simulink model "ES101A_DiagcMgrProxyX"  (R2013b)
settings: Solver=ode45  StartTime=0.0  StopTime=10.0  RelTol=1e-3
values from neighbouring files (symbols this model uses):
  DFTAGICNTR_CNT_U08 = DataDict.Constant    [ES101A_DiagcMgr_DataDict.m]
  DIAGCMGR_NTCINFOSTSTESTFAILD_CNT_U08 = DataDict.Constant    [ES101A_DiagcMgrProxyX_DataDict.m]    (also in ES101A_DiagcMgr_DataDict.m)
  DIAGCMGR_NTCINFOSTSTESTFAILDTHISIGNCYC_CNT_U08 = DataDict.Constant    [ES101A_DiagcMgr_DataDict.m]
  DIAGCMGR_NTCINFOSTSTESTNOTCMPLTHISIGNCYC_CNT_U08 = DataDict.Constant    [ES101A_DiagcMgrProxyX_DataDict.m]    (also in ES101A_DiagcMgr_DataDict.m)
  DiagcMgrFltResp = DataDict.Calibration    [ES101A_DiagcMgrProxyX_DataDict.m]    (also in ES101A_DiagcMgr_DataDict.m)
  DIAGCSTSDFTHWAG_CNT_U16 = DataDict.Constant    [ES101A_DiagcMgr_DataDict.m]
  DIAGCSTSDFTHWAGSERLCOMEXPRTVAL_CNT_U16 = DataDict.Constant    [ES101A_DiagcMgr_DataDict.m]
  DIAGCSTSDFTVEHSPD_CNT_U16 = DataDict.Constant    [ES101A_DiagcMgr_DataDict.m]
  DIAGCSTSININVAL_CNT_U16 = DataDict.Constant    [ES101A_DiagcMgrProxyX_DataDict.m]    (also in ES101A_DiagcMgr_DataDict.m)
  DIAGCSTSIVTR1INACTV_CNT_U16 = DataDict.Constant    [ES101A_DiagcMgr_DataDict.m]
  DIAGCSTSIVTR2INACTV_CNT_U16 = DataDict.Constant    [ES101A_DiagcMgr_DataDict.m]
  DIAGCSTSLIMDTPRFMNC_CNT_U16 = DataDict.Constant    [ES101A_DiagcMgr_DataDict.m]
  DIAGCSTSWHLIMBREJCTNDI_CNT_U16 = DataDict.Constant    [ES101A_DiagcMgr_DataDict.m]
  ELECGLBPRM_IVTRCNT_CNT_U08 = DataDict.ConfigParam    [ES101A_DiagcMgrProxyX_DataDict.m]    (also in ES101A_DiagcMgr_DataDict.m)
  MAXRAMPRATE_ULSPERSEC_F32 = DataDict.Constant    [ES101A_DiagcMgrProxyX_DataDict.m]    (also in ES101A_DiagcMgr_DataDict.m)
  MINRAMPRATE_ULSPERSEC_F32 = DataDict.Constant    [ES101A_DiagcMgrProxyX_DataDict.m]    (also in ES101A_DiagcMgr_DataDict.m)
  SCAMOTTQCMDTOONE_ULS_F32 = DataDict.Constant    [ES101A_DiagcMgrProxyX_DataDict.m]    (also in ES101A_DiagcMgr_DataDict.m)
  SCAMOTTQCMDTOZERO_ULS_F32 = DataDict.Constant    [ES101A_DiagcMgrProxyX_DataDict.m]    (also in ES101A_DiagcMgr_DataDict.m)
undefined symbols (not defined in the file or in its folder): ActvMotTqCmdSca, ActvRampRate, AgiCntr, DIAGCMGR_APPLIDXX_CNT_U08, DiagcMgrNtcMap, DiagcSts, NtcStInfo, Sts
libraries: simulink x21
(part 2 of 3)

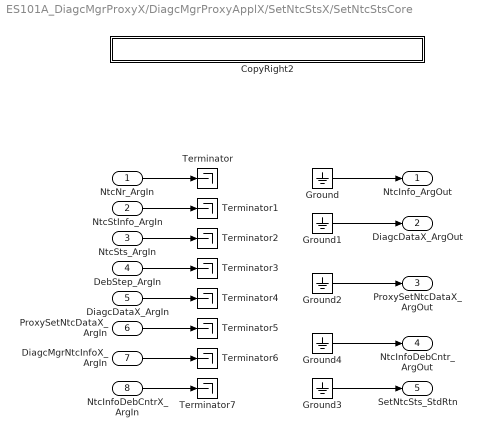
== system ES101A_DiagcMgrProxyX/DiagcMgrProxyApplX/SetNtcStsX/SetNtcStsCore ==
  NtcNr_ArgIn : Inport  OutDataTypeStr=Enum: NtcNr1
  NtcStInfo_ArgIn : Inport  Port=2
  NtcSts_ArgIn : Inport  Port=3
  DebStep_ArgIn : Inport  Port=4
  DiagcDataX_ArgIn : Inport  Port=5
  ProxySetNtcDataX_ArgIn : Inport  Port=6
  DiagcMgrNtcInfoX_ArgIn : Inport  Port=7
  NtcInfoDebCntrX_ArgIn : Inport  Port=8
  CopyRight2 : Subsystem  Description=|  mask(Copyright Information){none=on}
      | Copyright info block.                                               
      |                                                                     
      | Place copyright information at the top of every subsystem in design.
      mask prompts: none "No parameters"
      mask help: Place copyright information at the top of every subsystem in design.
      mask Display:
      | NxtrConf = 'Nexteer Confidential';
      | 
      | sys = bdroot; %handle for the current model ("system")
      | first = get_param(sys,'Created');
      | first = first(end-3:end);  %year is last four digits
      | 
      | last = get_param(sys,'LastModifiedDate');
      | if isempty(last)
      |     last = datestr(now,'yyyy');
      | else
      |     last = last(end-3:end);
      | end
      | 
      | if strcmp(first,last)
      |     fprintf('%s -- Copyright %s Nexteer',NxtrConf,first)
      | else
      |     fprintf('%s -- %s%s- %s Nexteer',NxtrConf,char(169),first,last)
      | end
  Ground{,1..4} (5 alike) : Ground
  Terminator{,1..7} (8 alike) : Terminator
  "NtcInfo_ArgOut " : Outport
  "DiagcDataX_ArgOut " : Outport  Port=2
  "ProxySetNtcDataX_ArgOut " : Outport  Port=3
  "NtcInfoDebCntr_ArgOut " : Outport  Port=4
  SetNtcSts_StdRtn : Outport  Port=5
  wires:
  NtcNr_ArgIn/1 -> Terminator/1
  NtcStInfo_ArgIn/1 -> Terminator1/1
  NtcSts_ArgIn/1 -> Terminator2/1
  DebStep_ArgIn/1 -> Terminator3/1
  DiagcDataX_ArgIn/1 -> Terminator4/1
  ProxySetNtcDataX_ArgIn/1 -> Terminator5/1
  DiagcMgrNtcInfoX_ArgIn/1 -> Terminator6/1
  NtcInfoDebCntrX_ArgIn/1 -> Terminator7/1
  Ground/1 -> "NtcInfo_ArgOut "/1
  Ground1/1 -> "DiagcDataX_ArgOut "/1
  Ground2/1 -> "ProxySetNtcDataX_ArgOut "/1
  Ground3/1 -> SetNtcSts_StdRtn/1
  Ground4/1 -> "NtcInfoDebCntr_ArgOut "/1

== system ES101A_DiagcMgrProxyX/DiagcMgrProxyApplX/DiagcMgrProxyApplXInit1/DiagcMgrIninCore/CopyRight2 ==

== system ES101A_DiagcMgrProxyX/DiagcMgrProxyApplX/DiagcMgrProxyApplXPer1/Clear All NTCs/CopyRight2 ==

== system ES101A_DiagcMgrProxyX/DiagcMgrProxyApplX/DiagcMgrProxyApplXPer1/Clear All NTCs/For Number of NTCs in NtcInfoAryX ==
  Number of Iterations : Inport
  Clear the NTCs that are active : Subsystem  RequirementInfo="{'linktype_rmi_doors' '0000c474 (/ESG Group/FDD Module Requirements/EA4 Specific/ES101A_DiagcMgr)' '#ES101A_298' 'true' 'REQ:  ES101A_298' '' ; 'linktype_rmi_doors' '0000c474 (/ESG Group/FDD Module Requirements/EA4 Specific/ES101A_DiagcMgr)' '#ES101A_185' 'true' 'REQ:  ES101A_185' '' ; 'linktype_rmi_doors' '0000c474 (/ESG Group/FDD Module Requirements/EA4 Specific/ES101A_DiagcMgr)' '#ES101A_256' 'true' 'REQ:  ES101A_256' '' ; 'linktype_rmi_doors' '0000c474 (/ESG Group/FDD Module Requirements/EA4 Specific/ES101A_DiagcMgr)' '#ES101A_255' 'true' 'REQ:  ES101A_255' '' ; 'linktype_rmi_doors' '0000c474 (/ESG Group/FDD Module Requirements/EA4 Specific/ES101A_DiagcMgr)' '#ES101A_254' 'true' 'REQ:  ES101A_254' '' ; 'linktype_rmi_doors' '0000c474 (/ESG Group/FDD Module Requirements/EA4 Specific/ES101A_DiagcMgr)' '#ES101A_297' 'true' 'REQ:  ES101A_297' '' ; 'linktype_rmi_doors' '0000c474 (/ESG Group/FDD Module Requirements/EA4 Specific/ES101A_DiagcMgr)' '#ES101A_305' 'true' 'REQ:  ES101A_305' '' } %GIDa_e344900f_fb8d_4798_8862_4b0202a8bbef"
  CopyRight2 : Subsystem  Description=|  mask(Copyright Information){none=on}
      | Copyright info block.                                               
      |                                                                     
      | Place copyright information at the top of every subsystem in design.
      mask prompts: none "No parameters"
      mask help: Place copyright information at the top of every subsystem in design.
      mask Display:
      | NxtrConf = 'Nexteer Confidential';
      | 
      | sys = bdroot; %handle for the current model ("system")
      | first = get_param(sys,'Created');
      | first = first(end-3:end);  %year is last four digits
      | 
      | last = get_param(sys,'LastModifiedDate');
      | if isempty(last)
      |     last = datestr(now,'yyyy');
      | else
      |     last = last(end-3:end);
      | end
      | 
      | if strcmp(first,last)
      |     fprintf('%s -- Copyright %s Nexteer',NxtrConf,first)
      | else
      |     fprintf('%s -- %s%s- %s Nexteer',NxtrConf,char(169),first,last)
      | end
  For Iterator : ForIterator  IterationSource=external  IterationLimit=255  IndexMode=Zero-based  IterationVariableDataType=int8
  wires:
  For Iterator/1 -> Clear the NTCs that are active/1(NtcInfoIdx)
  Number of Iterations/1 -> For Iterator/1

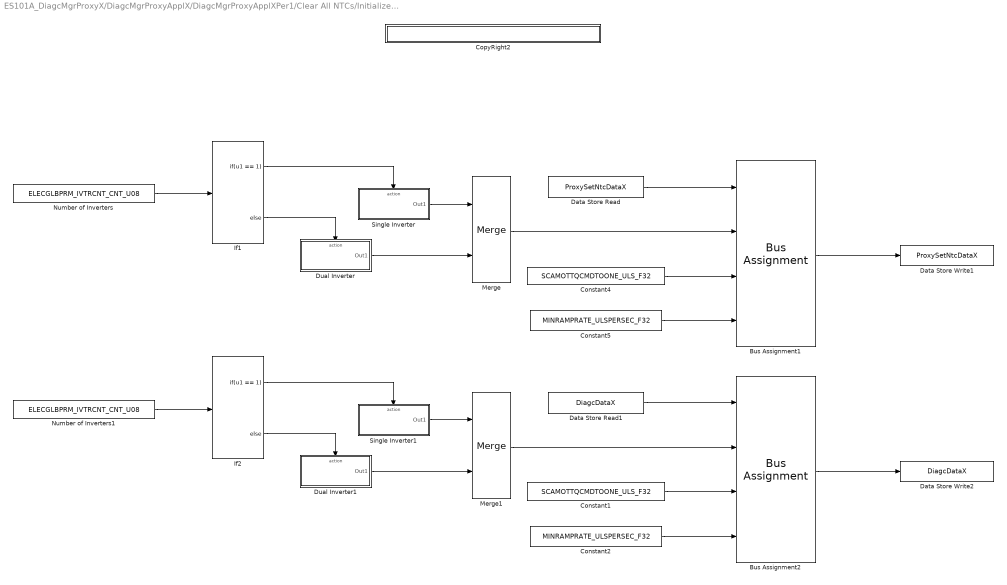
== system ES101A_DiagcMgrProxyX/DiagcMgrProxyApplX/DiagcMgrProxyApplXPer1/Clear All NTCs/Initialize Proxy SetNtc and DiagcData values ==
  Bus Assignment1 : BusAssignment  AssignedSignals=DiagcSts,ActvRampRate,ActvMotTqCmdSca
  Bus Assignment2 : BusAssignment  AssignedSignals=DiagcSts,ActvRampRate,ActvMotTqCmdSca
  Constant1 : Constant  Value=SCAMOTTQCMDTOONE_ULS_F32  OutDataTypeStr=single
  Constant2 : Constant  Value=MINRAMPRATE_ULSPERSEC_F32  OutDataTypeStr=single
  Constant4 : Constant  Value=SCAMOTTQCMDTOONE_ULS_F32  OutDataTypeStr=single
  Constant5 : Constant  Value=MINRAMPRATE_ULSPERSEC_F32  OutDataTypeStr=single
  CopyRight2 : Subsystem  Description=|  mask(Copyright Information){none=on}
      | Copyright info block.                                               
      |                                                                     
      | Place copyright information at the top of every subsystem in design.
      mask prompts: none "No parameters"
      mask help: Place copyright information at the top of every subsystem in design.
      mask Display:
      | NxtrConf = 'Nexteer Confidential';
      | 
      | sys = bdroot; %handle for the current model ("system")
      | first = get_param(sys,'Created');
      | first = first(end-3:end);  %year is last four digits
      | 
      | last = get_param(sys,'LastModifiedDate');
      | if isempty(last)
      |     last = datestr(now,'yyyy');
      | else
      |     last = last(end-3:end);
      | end
      | 
      | if strcmp(first,last)
      |     fprintf('%s -- Copyright %s Nexteer',NxtrConf,first)
      | else
      |     fprintf('%s -- %s%s- %s Nexteer',NxtrConf,char(169),first,last)
      | end
  Data Store Read : DataStoreRead  DataStoreName=ProxySetNtcDataX
  Data Store Read1 : DataStoreRead  DataStoreName=DiagcDataX
  Data Store Write1 : DataStoreWrite  DataStoreName=ProxySetNtcDataX
  Data Store Write2 : DataStoreWrite  DataStoreName=DiagcDataX
  Dual Inverter : Subsystem  TreatAsAtomicUnit=on
  Dual Inverter1 : Subsystem  TreatAsAtomicUnit=on
  If1 : If  IfExpression=u1 == 1
  If2 : If  IfExpression=u1 == 1
  Merge : Merge
  Merge1 : Merge
  Number of Inverters : Constant  Value=ELECGLBPRM_IVTRCNT_CNT_U08
  Number of Inverters1 : Constant  Value=ELECGLBPRM_IVTRCNT_CNT_U08
  Single Inverter : Subsystem  TreatAsAtomicUnit=on
  Single Inverter1 : Subsystem  TreatAsAtomicUnit=on
  wires:
  Data Store Read/1 -> Bus Assignment1/1
  Bus Assignment1/1 -> Data Store Write1/1
  Constant4/1 -> Bus Assignment1/3
  Constant5/1 -> Bus Assignment1/4
  Merge/1 -> Bus Assignment1/2
  If1/2 -> Dual Inverter/Action
  If1/1 -> Single Inverter/Action
  Number of Inverters/1 -> If1/1
  Dual Inverter/1(Out1) -> Merge/2
  Single Inverter/1(Out1) -> Merge/1
  Data Store Read1/1 -> Bus Assignment2/1
  Bus Assignment2/1 -> Data Store Write2/1
  Constant1/1 -> Bus Assignment2/3
  Constant2/1 -> Bus Assignment2/4
  Merge1/1 -> Bus Assignment2/2
  If2/2 -> Dual Inverter1/Action
  If2/1 -> Single Inverter1/Action
  Number of Inverters1/1 -> If2/1
  Dual Inverter1/1(Out1) -> Merge1/2
  Single Inverter1/1(Out1) -> Merge1/1

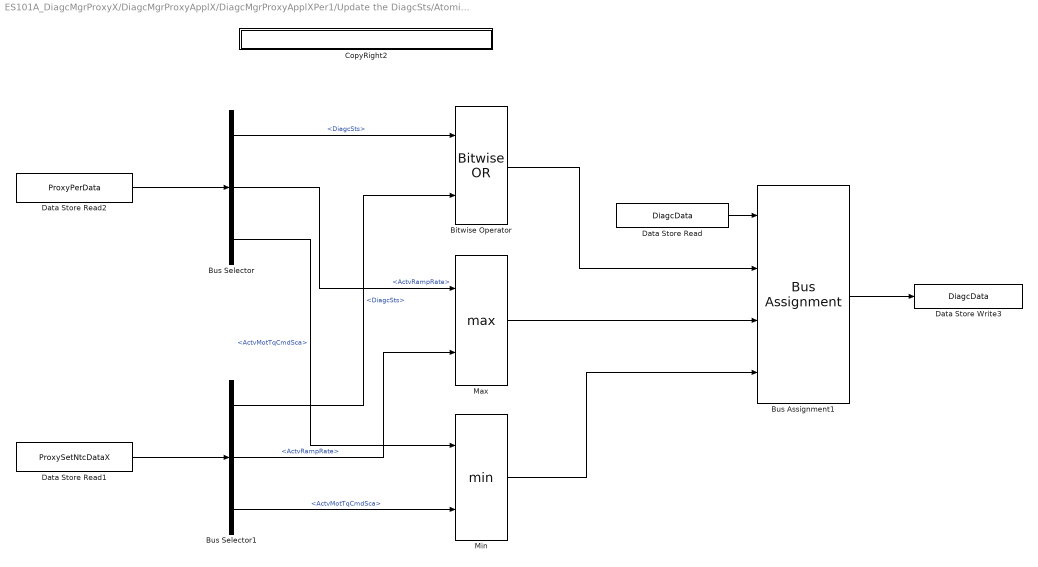
== system ES101A_DiagcMgrProxyX/DiagcMgrProxyApplX/DiagcMgrProxyApplXPer1/Update the DiagcSts/Atomic Section ==
  Bitwise Operator : simulink/Logic and Bit Operations/Bitwise Operator  logicop=OR  UseBitMask=off  NumInputPorts=2  BitMask=bin2dec('11011001')  BitMaskRealWorld=Stored Integer
  Bus Assignment1 : BusAssignment  AssignedSignals=DiagcSts,ActvRampRate,ActvMotTqCmdSca
  Bus Selector : BusSelector  OutputSignals=DiagcSts,ActvRampRate,ActvMotTqCmdSca
  Bus Selector1 : BusSelector  OutputSignals=DiagcSts,ActvRampRate,ActvMotTqCmdSca
  CopyRight2 : Subsystem  Description=|  mask(Copyright Information){none=on}
      | Copyright info block.                                               
      |                                                                     
      | Place copyright information at the top of every subsystem in design.
      mask prompts: none "No parameters"
      mask help: Place copyright information at the top of every subsystem in design.
      mask Display:
      | NxtrConf = 'Nexteer Confidential';
      | 
      | sys = bdroot; %handle for the current model ("system")
      | first = get_param(sys,'Created');
      | first = first(end-3:end);  %year is last four digits
      | 
      | last = get_param(sys,'LastModifiedDate');
      | if isempty(last)
      |     last = datestr(now,'yyyy');
      | else
      |     last = last(end-3:end);
      | end
      | 
      | if strcmp(first,last)
      |     fprintf('%s -- Copyright %s Nexteer',NxtrConf,first)
      | else
      |     fprintf('%s -- %s%s- %s Nexteer',NxtrConf,char(169),first,last)
      | end
  Data Store Read : DataStoreRead  DataStoreName=DiagcData  DataStoreElements=DiagcData
  Data Store Read1 : DataStoreRead  DataStoreName=ProxySetNtcDataX
  Data Store Read2 : DataStoreRead  DataStoreName=ProxyPerData
  Data Store Write3 : DataStoreWrite  DataStoreName=DiagcData  DataStoreElements=DiagcData
  Max : MinMax  Function=max  Inputs=2
  Min : MinMax  Inputs=2
  wires:
  Bus Selector/3 -> Min/1  "<ActvMotTqCmdSca>"
  Bus Selector1/3 -> Min/2  "<ActvMotTqCmdSca>"
  Bus Selector/2 -> Max/1  "<ActvRampRate>"
  Bus Selector1/2 -> Max/2  "<ActvRampRate>"
  Bus Selector/1 -> Bitwise Operator/1  "<DiagcSts>"
  Bus Selector1/1 -> Bitwise Operator/2  "<DiagcSts>"
  Data Store Read2/1 -> Bus Selector/1
  Data Store Read1/1 -> Bus Selector1/1
  Bus Assignment1/1 -> Data Store Write3/1
  Bitwise Operator/1 -> Bus Assignment1/2
  Max/1 -> Bus Assignment1/3
  Min/1 -> Bus Assignment1/4
  Data Store Read/1 -> Bus Assignment1/1

== system ES101A_DiagcMgrProxyX/DiagcMgrProxyApplX/DiagcMgrProxyApplXPer1/Update the DiagcSts/CopyRight2 ==

== system ES101A_DiagcMgrProxyX/DiagcMgrProxyApplX/DiagcMgrProxyApplXPer1/Update the DiagcSts/For Number of NTCs ==
  Number of Iterations : Inport
  Bus Selector2 : BusSelector  OutputSignals=Sts
  CopyRight2 : Subsystem  Description=|  mask(Copyright Information){none=on}
      | Copyright info block.                                               
      |                                                                     
      | Place copyright information at the top of every subsystem in design.
      mask prompts: none "No parameters"
      mask help: Place copyright information at the top of every subsystem in design.
      mask Display:
      | NxtrConf = 'Nexteer Confidential';
      | 
      | sys = bdroot; %handle for the current model ("system")
      | first = get_param(sys,'Created');
      | first = first(end-3:end);  %year is last four digits
      | 
      | last = get_param(sys,'LastModifiedDate');
      | if isempty(last)
      |     last = datestr(now,'yyyy');
      | else
      |     last = last(end-3:end);
      | end
      | 
      | if strcmp(first,last)
      |     fprintf('%s -- Copyright %s Nexteer',NxtrConf,first)
      | else
      |     fprintf('%s -- %s%s- %s Nexteer',NxtrConf,char(169),first,last)
      | end
  Data Store Read1 : DataStoreRead  DataStoreName=NtcNrAryApplX
  Data Store Read2 : DataStoreRead  DataStoreName=DiagcMgrNtcInfoXAry
  For Iterator : ForIterator  IterationSource=external  IndexMode=Zero-based
  Selector1 : Selector  IndexMode=Zero-based  InputPortWidth=1  IndexOptions=Index vector (port)  Indices=[1 3]  OutputSizes=1
  Selector2 : Selector  IndexMode=Zero-based  InputPortWidth=1  IndexOptions=Index vector (port)  Indices=[1 3]  OutputSizes=1
  Update DiagcSts and Ramp Response : Subsystem  TreatAsAtomicUnit=on
  wires:
  Number of Iterations/1 -> For Iterator/1
  For Iterator/1 -> Selector2/2, Selector1/2
  Selector1/1 -> Bus Selector2/1
  Data Store Read2/1 -> Selector1/1
  Bus Selector2/1 -> Update DiagcSts and Ramp Response/1(Sts)  "<Sts>"
  Data Store Read1/1 -> Selector2/1
  Selector2/1 -> Update DiagcSts and Ramp Response/2(NtcNr)

== system ES101A_DiagcMgrProxyX/DiagcMgrProxyApplX/DiagcMgrProxyApplXPer1/Update the DiagcSts/Initialize Proxy Per values ==
  Bus Assignment1 : BusAssignment  AssignedSignals=DiagcSts,ActvRampRate,ActvMotTqCmdSca
  Constant4 : Constant  Value=SCAMOTTQCMDTOONE_ULS_F32  OutDataTypeStr=single
  Constant5 : Constant  Value=MINRAMPRATE_ULSPERSEC_F32  OutDataTypeStr=single
  CopyRight2 : Subsystem  Description=|  mask(Copyright Information){none=on}
      | Copyright info block.                                               
      |                                                                     
      | Place copyright information at the top of every subsystem in design.
      mask prompts: none "No parameters"
      mask help: Place copyright information at the top of every subsystem in design.
      mask Display:
      | NxtrConf = 'Nexteer Confidential';
      | 
      | sys = bdroot; %handle for the current model ("system")
      | first = get_param(sys,'Created');
      | first = first(end-3:end);  %year is last four digits
      | 
      | last = get_param(sys,'LastModifiedDate');
      | if isempty(last)
      |     last = datestr(now,'yyyy');
      | else
      |     last = last(end-3:end);
      | end
      | 
      | if strcmp(first,last)
      |     fprintf('%s -- Copyright %s Nexteer',NxtrConf,first)
      | else
      |     fprintf('%s -- %s%s- %s Nexteer',NxtrConf,char(169),first,last)
      | end
  Data Store Read : DataStoreRead  DataStoreName=ProxyPerData
  Data Store Write1 : DataStoreWrite  DataStoreName=ProxyPerData
  Dual Inverter : Subsystem  TreatAsAtomicUnit=on
  If1 : If  IfExpression=u1 == 1
  Merge : Merge
  Number of Inverters : Constant  Value=ELECGLBPRM_IVTRCNT_CNT_U08
  Single Inverter : Subsystem  TreatAsAtomicUnit=on
  wires:
  Data Store Read/1 -> Bus Assignment1/1
  Bus Assignment1/1 -> Data Store Write1/1
  Constant4/1 -> Bus Assignment1/3
  Constant5/1 -> Bus Assignment1/4
  Merge/1 -> Bus Assignment1/2
  If1/2 -> Dual Inverter/Action
  If1/1 -> Single Inverter/Action
  Number of Inverters/1 -> If1/1
  Dual Inverter/1(Out1) -> Merge/2
  Single Inverter/1(Out1) -> Merge/1

== system ES101A_DiagcMgrProxyX/DiagcMgrProxyApplX/DiagcMgrProxyApplXPer1/Update the DiagcSts/Initialize Proxy SetNtc values ==
  Bus Assignment1 : BusAssignment  AssignedSignals=DiagcSts,ActvRampRate,ActvMotTqCmdSca
  Constant4 : Constant  Value=SCAMOTTQCMDTOONE_ULS_F32  OutDataTypeStr=single
  Constant5 : Constant  Value=MINRAMPRATE_ULSPERSEC_F32  OutDataTypeStr=single
  CopyRight2 : Subsystem  Description=|  mask(Copyright Information){none=on}
      | Copyright info block.                                               
      |                                                                     
      | Place copyright information at the top of every subsystem in design.
      mask prompts: none "No parameters"
      mask help: Place copyright information at the top of every subsystem in design.
      mask Display:
      | NxtrConf = 'Nexteer Confidential';
      | 
      | sys = bdroot; %handle for the current model ("system")
      | first = get_param(sys,'Created');
      | first = first(end-3:end);  %year is last four digits
      | 
      | last = get_param(sys,'LastModifiedDate');
      | if isempty(last)
      |     last = datestr(now,'yyyy');
      | else
      |     last = last(end-3:end);
      | end
      | 
      | if strcmp(first,last)
      |     fprintf('%s -- Copyright %s Nexteer',NxtrConf,first)
      | else
      |     fprintf('%s -- %s%s- %s Nexteer',NxtrConf,char(169),first,last)
      | end
  Data Store Read : DataStoreRead  DataStoreName=ProxySetNtcDataX
  Data Store Write1 : DataStoreWrite  DataStoreName=ProxySetNtcDataX
  Dual Inverter : Subsystem  TreatAsAtomicUnit=on
  If1 : If  IfExpression=u1 == 1
  Merge : Merge
  Number of Inverters : Constant  Value=ELECGLBPRM_IVTRCNT_CNT_U08
  Single Inverter : Subsystem  TreatAsAtomicUnit=on
  wires:
  Data Store Read/1 -> Bus Assignment1/1
  Bus Assignment1/1 -> Data Store Write1/1
  Constant4/1 -> Bus Assignment1/3
  Constant5/1 -> Bus Assignment1/4
  Merge/1 -> Bus Assignment1/2
  If1/2 -> Dual Inverter/Action
  If1/1 -> Single Inverter/Action
  Number of Inverters/1 -> If1/1
  Dual Inverter/1(Out1) -> Merge/2
  Single Inverter/1(Out1) -> Merge/1

== system ES101A_DiagcMgrProxyX/DiagcMgrProxyApplX/GetNtcActvX/GetNtcActvCore/CopyRight2 ==

== system ES101A_DiagcMgrProxyX/DiagcMgrProxyApplX/GetNtcQlfrStsX/GetNtcQlfrStsCore/CopyRight2 ==

== system ES101A_DiagcMgrProxyX/DiagcMgrProxyApplX/GetNtcStsX/GetNtcStsCore/CopyRight2 ==

== system ES101A_DiagcMgrProxyX/DiagcMgrProxyApplX/SetNtcStsX/SetNtcStsCore/CopyRight2 ==

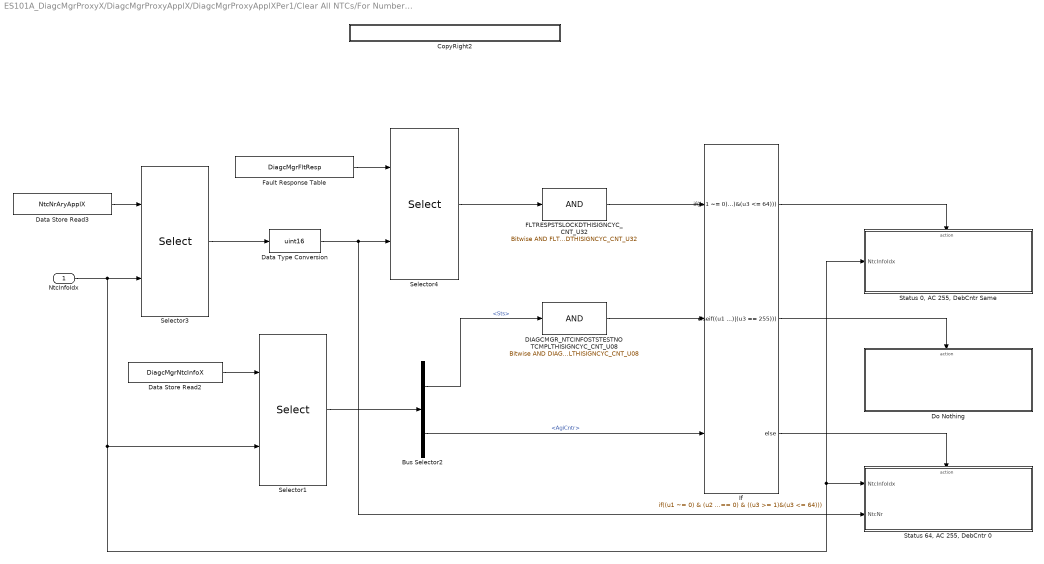
== system ES101A_DiagcMgrProxyX/DiagcMgrProxyApplX/DiagcMgrProxyApplXPer1/Clear All NTCs/For Number of NTCs in NtcInfoAryX/Clear the NTCs that are active ==
  NtcInfoIdx : Inport
  Bus Selector2 : BusSelector  OutputSignals=Sts,AgiCntr
  CopyRight2 : Subsystem  Description=|  mask(Copyright Information){none=on}
      | Copyright info block.                                               
      |                                                                     
      | Place copyright information at the top of every subsystem in design.
      mask prompts: none "No parameters"
      mask help: Place copyright information at the top of every subsystem in design.
      mask Display:
      | NxtrConf = 'Nexteer Confidential';
      | 
      | sys = bdroot; %handle for the current model ("system")
      | first = get_param(sys,'Created');
      | first = first(end-3:end);  %year is last four digits
      | 
      | last = get_param(sys,'LastModifiedDate');
      | if isempty(last)
      |     last = datestr(now,'yyyy');
      | else
      |     last = last(end-3:end);
      | end
      | 
      | if strcmp(first,last)
      |     fprintf('%s -- Copyright %s Nexteer',NxtrConf,first)
      | else
      |     fprintf('%s -- %s%s- %s Nexteer',NxtrConf,char(169),first,last)
      | end
  DIAGCMGR_NTCINFOSTSTESTNOTCMPLTHISIGNCYC_CNT_U08 : simulink/Logic and Bit Operations/Bitwise Operator  logicop=AND  UseBitMask=on  BitMask=DIAGCMGR_NTCINFOSTSTESTNOTCMPLTHISIGNCYC_CNT_U08  BitMaskRealWorld=Stored Integer
  Data Store Read2 : DataStoreRead  DataStoreName=DiagcMgrNtcInfoX
  Data Store Read3 : DataStoreRead  DataStoreName=NtcNrAryApplX
  Data Type Conversion : DataTypeConversion  OutDataTypeStr=uint16
  Do Nothing : Subsystem  TreatAsAtomicUnit=on
  FLTRESPSTSLOCKDTHISIGNCYC_CNT_U32 : simulink/Logic and Bit Operations/Bitwise Operator  RequirementInfo={} %GIDa_3c8fd334_aaa1_4aae_92b3_7b41709ff7dc  logicop=AND  UseBitMask=on  BitMask=FLTRESPSTSLOCKDTHISIGNCYC_CNT_U32  BitMaskRealWorld=Stored Integer
  Fault Response Table : Constant  Value=DiagcMgrFltResp
  If : If  NumInputs=3  IfExpression=(u1 ~= 0) & (u2 == 0) & ((u3 >= 1)&(u3 <= 64))  ElseIfExpressions=(u1 ~= 0) & (u2 == 0) & ((u3 == 0)|(u3 == 255))
  Selector1 : Selector  IndexMode=Zero-based  InputPortWidth=512  IndexOptions=Index vector (port)  Indices=[1 3]  OutputSizes=1
  Selector3 : Selector  IndexMode=Zero-based  InputPortWidth=22  IndexOptions=Index vector (port)  Indices=[1 3]  OutputSizes=1
  Selector4 : Selector  IndexMode=Zero-based  InputPortWidth=512  IndexOptions=Index vector (port)  Indices=[1 3]  OutputSizes=1
  "Status 0, AC 255, DebCntr Same" : Subsystem  TreatAsAtomicUnit=on
  "Status 64, AC 255, DebCntr 0" : Subsystem
  wires:
  Data Store Read3/1 -> Selector3/1
  Selector3/1 -> Data Type Conversion/1
  Fault Response Table/1 -> Selector4/1
  Selector4/1 -> FLTRESPSTSLOCKDTHISIGNCYC_CNT_U32/1
  FLTRESPSTSLOCKDTHISIGNCYC_CNT_U32/1 -> If/1
  Selector1/1 -> Bus Selector2/1
  Data Store Read2/1 -> Selector1/1
  Bus Selector2/1 -> DIAGCMGR_NTCINFOSTSTESTNOTCMPLTHISIGNCYC_CNT_U08/1  "<Sts>"
  Bus Selector2/2 -> If/3  "<AgiCntr>"
  DIAGCMGR_NTCINFOSTSTESTNOTCMPLTHISIGNCYC_CNT_U08/1 -> If/2
  Data Type Conversion/1 -> "Status 64, AC 255, DebCntr 0"/2(NtcNr), Selector4/2
  NtcInfoIdx/1 -> Selector3/2, "Status 0, AC 255, DebCntr Same"/1(NtcInfoIdx), "Status 64, AC 255, DebCntr 0"/1(NtcInfoIdx), Selector1/2
  If/3 -> "Status 64, AC 255, DebCntr 0"/Action
  If/2 -> Do Nothing/Action
  If/1 -> "Status 0, AC 255, DebCntr Same"/Action

== system ES101A_DiagcMgrProxyX/DiagcMgrProxyApplX/DiagcMgrProxyApplXPer1/Clear All NTCs/For Number of NTCs in NtcInfoAryX/CopyRight2 ==

== system ES101A_DiagcMgrProxyX/DiagcMgrProxyApplX/DiagcMgrProxyApplXPer1/Clear All NTCs/Initialize Proxy SetNtc and DiagcData values/CopyRight2 ==

== system ES101A_DiagcMgrProxyX/DiagcMgrProxyApplX/DiagcMgrProxyApplXPer1/Clear All NTCs/Initialize Proxy SetNtc and DiagcData values/Dual Inverter ==
  Action Port : ActionPort
  CopyRight2 : Subsystem  Description=|  mask(Copyright Information){none=on}
      | Copyright info block.                                               
      |                                                                     
      | Place copyright information at the top of every subsystem in design.
      mask prompts: none "No parameters"
      mask help: Place copyright information at the top of every subsystem in design.
      mask Display:
      | NxtrConf = 'Nexteer Confidential';
      | 
      | sys = bdroot; %handle for the current model ("system")
      | first = get_param(sys,'Created');
      | first = first(end-3:end);  %year is last four digits
      | 
      | last = get_param(sys,'LastModifiedDate');
      | if isempty(last)
      |     last = datestr(now,'yyyy');
      | else
      |     last = last(end-3:end);
      | end
      | 
      | if strcmp(first,last)
      |     fprintf('%s -- Copyright %s Nexteer',NxtrConf,first)
      | else
      |     fprintf('%s -- %s%s- %s Nexteer',NxtrConf,char(169),first,last)
      | end
  Inverter 2 Inactive : Constant  Value=0  OutDataTypeStr=uint16
  Out1 : Outport
  wires:
  Inverter 2 Inactive/1 -> Out1/1

== system ES101A_DiagcMgrProxyX/DiagcMgrProxyApplX/DiagcMgrProxyApplXPer1/Clear All NTCs/Initialize Proxy SetNtc and DiagcData values/Dual Inverter1 ==
  Action Port : ActionPort
  CopyRight2 : Subsystem  Description=|  mask(Copyright Information){none=on}
      | Copyright info block.                                               
      |                                                                     
      | Place copyright information at the top of every subsystem in design.
      mask prompts: none "No parameters"
      mask help: Place copyright information at the top of every subsystem in design.
      mask Display:
      | NxtrConf = 'Nexteer Confidential';
      | 
      | sys = bdroot; %handle for the current model ("system")
      | first = get_param(sys,'Created');
      | first = first(end-3:end);  %year is last four digits
      | 
      | last = get_param(sys,'LastModifiedDate');
      | if isempty(last)
      |     last = datestr(now,'yyyy');
      | else
      |     last = last(end-3:end);
      | end
      | 
      | if strcmp(first,last)
      |     fprintf('%s -- Copyright %s Nexteer',NxtrConf,first)
      | else
      |     fprintf('%s -- %s%s- %s Nexteer',NxtrConf,char(169),first,last)
      | end
  Inverter 2 Inactive : Constant  Value=0  OutDataTypeStr=uint16
  Out1 : Outport
  wires:
  Inverter 2 Inactive/1 -> Out1/1

== system ES101A_DiagcMgrProxyX/DiagcMgrProxyApplX/DiagcMgrProxyApplXPer1/Clear All NTCs/Initialize Proxy SetNtc and DiagcData values/Single Inverter ==
  Action Port : ActionPort
  CopyRight2 : Subsystem  Description=|  mask(Copyright Information){none=on}
      | Copyright info block.                                               
      |                                                                     
      | Place copyright information at the top of every subsystem in design.
      mask prompts: none "No parameters"
      mask help: Place copyright information at the top of every subsystem in design.
      mask Display:
      | NxtrConf = 'Nexteer Confidential';
      | 
      | sys = bdroot; %handle for the current model ("system")
      | first = get_param(sys,'Created');
      | first = first(end-3:end);  %year is last four digits
      | 
      | last = get_param(sys,'LastModifiedDate');
      | if isempty(last)
      |     last = datestr(now,'yyyy');
      | else
      |     last = last(end-3:end);
      | end
      | 
      | if strcmp(first,last)
      |     fprintf('%s -- Copyright %s Nexteer',NxtrConf,first)
      | else
      |     fprintf('%s -- %s%s- %s Nexteer',NxtrConf,char(169),first,last)
      | end
  Inverter 2 Inactive : Constant  Value=DIAGCSTSIVTR2INACTV_CNT_U16  OutDataTypeStr=uint16
  Out1 : Outport
  wires:
  Inverter 2 Inactive/1 -> Out1/1

== system ES101A_DiagcMgrProxyX/DiagcMgrProxyApplX/DiagcMgrProxyApplXPer1/Clear All NTCs/Initialize Proxy SetNtc and DiagcData values/Single Inverter1 ==
  Action Port : ActionPort
  CopyRight2 : Subsystem  Description=|  mask(Copyright Information){none=on}
      | Copyright info block.                                               
      |                                                                     
      | Place copyright information at the top of every subsystem in design.
      mask prompts: none "No parameters"
      mask help: Place copyright information at the top of every subsystem in design.
      mask Display:
      | NxtrConf = 'Nexteer Confidential';
      | 
      | sys = bdroot; %handle for the current model ("system")
      | first = get_param(sys,'Created');
      | first = first(end-3:end);  %year is last four digits
      | 
      | last = get_param(sys,'LastModifiedDate');
      | if isempty(last)
      |     last = datestr(now,'yyyy');
      | else
      |     last = last(end-3:end);
      | end
      | 
      | if strcmp(first,last)
      |     fprintf('%s -- Copyright %s Nexteer',NxtrConf,first)
      | else
      |     fprintf('%s -- %s%s- %s Nexteer',NxtrConf,char(169),first,last)
      | end
  Inverter 2 Inactive : Constant  Value=DIAGCSTSIVTR2INACTV_CNT_U16  OutDataTypeStr=uint16
  Out1 : Outport
  wires:
  Inverter 2 Inactive/1 -> Out1/1

== system ES101A_DiagcMgrProxyX/DiagcMgrProxyApplX/DiagcMgrProxyApplXPer1/Update the DiagcSts/Atomic Section/CopyRight2 ==

== system ES101A_DiagcMgrProxyX/DiagcMgrProxyApplX/DiagcMgrProxyApplXPer1/Update the DiagcSts/For Number of NTCs/CopyRight2 ==

== system ES101A_DiagcMgrProxyX/DiagcMgrProxyApplX/DiagcMgrProxyApplXPer1/Update the DiagcSts/For Number of NTCs/Update DiagcSts and Ramp Response ==
  Sts : Inport
  NtcNr : Inport  Port=2
  Bitwise Operator : simulink/Logic and Bit Operations/Bitwise Operator  logicop=AND  UseBitMask=off  NumInputPorts=2  BitMask=bin2dec('11011001')  BitMaskRealWorld=Stored Integer
  Bitwise Operator1 : simulink/Logic and Bit Operations/Bitwise Operator  logicop=AND  UseBitMask=off  NumInputPorts=2  BitMask=bin2dec('11011001')  BitMaskRealWorld=Stored Integer
  CopyRight2 : Subsystem  Description=|  mask(Copyright Information){none=on}
      | Copyright info block.                                               
      |                                                                     
      | Place copyright information at the top of every subsystem in design.
      mask prompts: none "No parameters"
      mask help: Place copyright information at the top of every subsystem in design.
      mask Display:
      | NxtrConf = 'Nexteer Confidential';
      | 
      | sys = bdroot; %handle for the current model ("system")
      | first = get_param(sys,'Created');
      | first = first(end-3:end);  %year is last four digits
      | 
      | last = get_param(sys,'LastModifiedDate');
      | if isempty(last)
      |     last = datestr(now,'yyyy');
      | else
      |     last = last(end-3:end);
      | end
      | 
      | if strcmp(first,last)
      |     fprintf('%s -- Copyright %s Nexteer',NxtrConf,first)
      | else
      |     fprintf('%s -- %s%s- %s Nexteer',NxtrConf,char(169),first,last)
      | end
  Do Nothing : Subsystem  TreatAsAtomicUnit=on
  If : If  IfExpression=u1 == 1
  Logical Operator : Logic  AllPortsSameDT=off  OutDataTypeStr=boolean
  NTC Test Failed Bit : Constant  Value=DIAGCMGR_NTCINFOSTSTESTFAILD_CNT_U08
  NTC Test Failed This Ignition Cycle Bit : Constant  Value=DIAGCMGR_NTCINFOSTSTESTFAILDTHISIGNCYC_CNT_U08
  Update Latest Values : Subsystem  TreatAsAtomicUnit=on
  wires:
  NtcNr/1 -> Update Latest Values/1(NtcNr)
  NTC Test Failed Bit/1 -> Bitwise Operator/1
  If/2 -> Do Nothing/Action
  If/1 -> Update Latest Values/Action
  NTC Test Failed This Ignition Cycle Bit/1 -> Bitwise Operator1/1
  Sts/1 -> Bitwise Operator/2, Bitwise Operator1/2
  Logical Operator/1 -> If/1
  Bitwise Operator1/1 -> Logical Operator/1
  Bitwise Operator/1 -> Logical Operator/2

== system ES101A_DiagcMgrProxyX/DiagcMgrProxyApplX/DiagcMgrProxyApplXPer1/Update the DiagcSts/Initialize Proxy Per values/CopyRight2 ==

== system ES101A_DiagcMgrProxyX/DiagcMgrProxyApplX/DiagcMgrProxyApplXPer1/Update the DiagcSts/Initialize Proxy Per values/Dual Inverter ==
  Action Port : ActionPort
  CopyRight2 : Subsystem  Description=|  mask(Copyright Information){none=on}
      | Copyright info block.                                               
      |                                                                     
      | Place copyright information at the top of every subsystem in design.
      mask prompts: none "No parameters"
      mask help: Place copyright information at the top of every subsystem in design.
      mask Display:
      | NxtrConf = 'Nexteer Confidential';
      | 
      | sys = bdroot; %handle for the current model ("system")
      | first = get_param(sys,'Created');
      | first = first(end-3:end);  %year is last four digits
      | 
      | last = get_param(sys,'LastModifiedDate');
      | if isempty(last)
      |     last = datestr(now,'yyyy');
      | else
      |     last = last(end-3:end);
      | end
      | 
      | if strcmp(first,last)
      |     fprintf('%s -- Copyright %s Nexteer',NxtrConf,first)
      | else
      |     fprintf('%s -- %s%s- %s Nexteer',NxtrConf,char(169),first,last)
      | end
  Inverter 2 Inactive : Constant  Value=DIAGCSTSININVAL_CNT_U16  OutDataTypeStr=uint16
  Out1 : Outport
  wires:
  Inverter 2 Inactive/1 -> Out1/1

== system ES101A_DiagcMgrProxyX/DiagcMgrProxyApplX/DiagcMgrProxyApplXPer1/Update the DiagcSts/Initialize Proxy Per values/Single Inverter ==
  Action Port : ActionPort
  CopyRight2 : Subsystem  Description=|  mask(Copyright Information){none=on}
      | Copyright info block.                                               
      |                                                                     
      | Place copyright information at the top of every subsystem in design.
      mask prompts: none "No parameters"
      mask help: Place copyright information at the top of every subsystem in design.
      mask Display:
      | NxtrConf = 'Nexteer Confidential';
      | 
      | sys = bdroot; %handle for the current model ("system")
      | first = get_param(sys,'Created');
      | first = first(end-3:end);  %year is last four digits
      | 
      | last = get_param(sys,'LastModifiedDate');
      | if isempty(last)
      |     last = datestr(now,'yyyy');
      | else
      |     last = last(end-3:end);
      | end
      | 
      | if strcmp(first,last)
      |     fprintf('%s -- Copyright %s Nexteer',NxtrConf,first)
      | else
      |     fprintf('%s -- %s%s- %s Nexteer',NxtrConf,char(169),first,last)
      | end
  Inverter 2 Inactive : Constant  Value=DIAGCSTSIVTR2INACTV_CNT_U16  OutDataTypeStr=uint16
  Out1 : Outport
  wires:
  Inverter 2 Inactive/1 -> Out1/1

== system ES101A_DiagcMgrProxyX/DiagcMgrProxyApplX/DiagcMgrProxyApplXPer1/Update the DiagcSts/Initialize Proxy SetNtc values/CopyRight2 ==

== system ES101A_DiagcMgrProxyX/DiagcMgrProxyApplX/DiagcMgrProxyApplXPer1/Update the DiagcSts/Initialize Proxy SetNtc values/Dual Inverter ==
  Action Port : ActionPort
  CopyRight2 : Subsystem  Description=|  mask(Copyright Information){none=on}
      | Copyright info block.                                               
      |                                                                     
      | Place copyright information at the top of every subsystem in design.
      mask prompts: none "No parameters"
      mask help: Place copyright information at the top of every subsystem in design.
      mask Display:
      | NxtrConf = 'Nexteer Confidential';
      | 
      | sys = bdroot; %handle for the current model ("system")
      | first = get_param(sys,'Created');
      | first = first(end-3:end);  %year is last four digits
      | 
      | last = get_param(sys,'LastModifiedDate');
      | if isempty(last)
      |     last = datestr(now,'yyyy');
      | else
      |     last = last(end-3:end);
      | end
      | 
      | if strcmp(first,last)
      |     fprintf('%s -- Copyright %s Nexteer',NxtrConf,first)
      | else
      |     fprintf('%s -- %s%s- %s Nexteer',NxtrConf,char(169),first,last)
      | end
  Inverter 2 Inactive : Constant  Value=DIAGCSTSININVAL_CNT_U16  OutDataTypeStr=uint16
  Out1 : Outport
  wires:
  Inverter 2 Inactive/1 -> Out1/1

== system ES101A_DiagcMgrProxyX/DiagcMgrProxyApplX/DiagcMgrProxyApplXPer1/Update the DiagcSts/Initialize Proxy SetNtc values/Single Inverter ==
  Action Port : ActionPort
  CopyRight2 : Subsystem  Description=|  mask(Copyright Information){none=on}
      | Copyright info block.                                               
      |                                                                     
      | Place copyright information at the top of every subsystem in design.
      mask prompts: none "No parameters"
      mask help: Place copyright information at the top of every subsystem in design.
      mask Display:
      | NxtrConf = 'Nexteer Confidential';
      | 
      | sys = bdroot; %handle for the current model ("system")
      | first = get_param(sys,'Created');
      | first = first(end-3:end);  %year is last four digits
      | 
      | last = get_param(sys,'LastModifiedDate');
      | if isempty(last)
      |     last = datestr(now,'yyyy');
      | else
      |     last = last(end-3:end);
      | end
      | 
      | if strcmp(first,last)
      |     fprintf('%s -- Copyright %s Nexteer',NxtrConf,first)
      | else
      |     fprintf('%s -- %s%s- %s Nexteer',NxtrConf,char(169),first,last)
      | end
  Inverter 2 Inactive : Constant  Value=DIAGCSTSIVTR2INACTV_CNT_U16  OutDataTypeStr=uint16
  Out1 : Outport
  wires:
  Inverter 2 Inactive/1 -> Out1/1

== system ES101A_DiagcMgrProxyX/DiagcMgrProxyApplX/DiagcMgrProxyApplXPer1/Clear All NTCs/For Number of NTCs in NtcInfoAryX/Clear the NTCs that are active/CopyRight2 ==

== system ES101A_DiagcMgrProxyX/DiagcMgrProxyApplX/DiagcMgrProxyApplXPer1/Clear All NTCs/For Number of NTCs in NtcInfoAryX/Clear the NTCs that are active/Do Nothing ==
  Action Port : ActionPort  ActionType=elseif
  CopyRight2 : Subsystem  Description=|  mask(Copyright Information){none=on}
      | Copyright info block.                                               
      |                                                                     
      | Place copyright information at the top of every subsystem in design.
      mask prompts: none "No parameters"
      mask help: Place copyright information at the top of every subsystem in design.
      mask Display:
      | NxtrConf = 'Nexteer Confidential';
      | 
      | sys = bdroot; %handle for the current model ("system")
      | first = get_param(sys,'Created');
      | first = first(end-3:end);  %year is last four digits
      | 
      | last = get_param(sys,'LastModifiedDate');
      | if isempty(last)
      |     last = datestr(now,'yyyy');
      | else
      |     last = last(end-3:end);
      | end
      | 
      | if strcmp(first,last)
      |     fprintf('%s -- Copyright %s Nexteer',NxtrConf,first)
      | else
      |     fprintf('%s -- %s%s- %s Nexteer',NxtrConf,char(169),first,last)
      | end

== system ES101A_DiagcMgrProxyX/DiagcMgrProxyApplX/DiagcMgrProxyApplXPer1/Clear All NTCs/For Number of NTCs in NtcInfoAryX/Clear the NTCs that are active/Status 0, AC 255, DebCntr Same ==
  NtcInfoIdx : Inport
  Action Port : ActionPort  ActionType=then
  Assignment : Assignment  IndexMode=Zero-based  IndexOptions=Index vector (port)  Indices=1  OutputSizes=1
  Bus Assignment4 : BusAssignment  AssignedSignals=Sts,NtcStInfo,AgiCntr
  Constant1 : Constant  Value=0  OutDataTypeStr=int16
  Constant3 : Constant  Value=0
  Constant4 : Constant  Value=DFTAGICNTR_CNT_U08  OutDataTypeStr=int16
  Data Store Read : DataStoreRead  DataStoreName=DiagcMgrNtcInfoXAry
  Data Store Read1 : DataStoreRead  DataStoreName=DiagcMgrNtcInfoXAry
  Data Store Write2 : DataStoreWrite  DataStoreName=DiagcMgrNtcInfoXAry
  Selector : Selector  IndexMode=Zero-based  InputPortWidth=22  IndexOptions=Index vector (port)  Indices=[1 3]  OutputSizes=1
  wires:
  Data Store Read1/1 -> Assignment/1
  Selector/1 -> Bus Assignment4/1
  NtcInfoIdx/1 -> Assignment/3, Selector/2
  Data Store Read/1 -> Selector/1
  Assignment/1 -> Data Store Write2/1
  Constant1/1 -> Bus Assignment4/3
  Constant4/1 -> Bus Assignment4/4
  Bus Assignment4/1 -> Assignment/2
  Constant3/1 -> Bus Assignment4/2

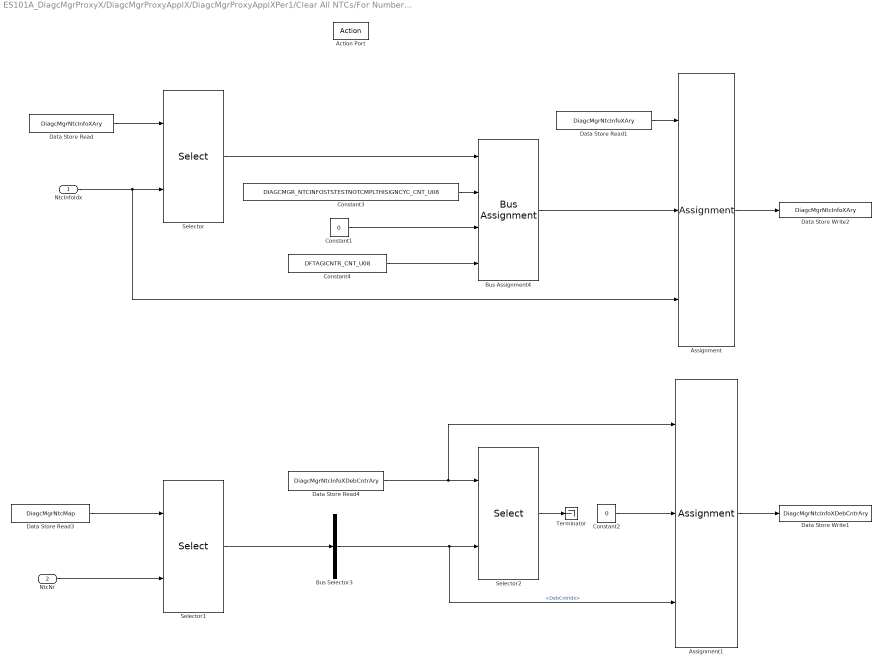
== system ES101A_DiagcMgrProxyX/DiagcMgrProxyApplX/DiagcMgrProxyApplXPer1/Clear All NTCs/For Number of NTCs in NtcInfoAryX/Clear the NTCs that are active/Status 64, AC 255, DebCntr 0 ==
  NtcInfoIdx : Inport
  NtcNr : Inport  Port=2
  Action Port : ActionPort  ActionType=else
  Assignment : Assignment  IndexMode=Zero-based  IndexOptions=Index vector (port)  Indices=1  OutputSizes=1
  Assignment1 : Assignment  IndexMode=Zero-based  IndexOptions=Index vector (port)  Indices=1  OutputSizes=1
  Bus Assignment4 : BusAssignment  AssignedSignals=Sts,NtcStInfo,AgiCntr
  Bus Selector3 : BusSelector  OutputSignals=DebCntrIdx
  Constant1 : Constant  Value=0  OutDataTypeStr=int16
  Constant2 : Constant  Value=0  OutDataTypeStr=int16
  Constant3 : Constant  Value=DIAGCMGR_NTCINFOSTSTESTNOTCMPLTHISIGNCYC_CNT_U08
  Constant4 : Constant  Value=DFTAGICNTR_CNT_U08  OutDataTypeStr=int16
  Data Store Read : DataStoreRead  DataStoreName=DiagcMgrNtcInfoXAry
  Data Store Read1 : DataStoreRead  DataStoreName=DiagcMgrNtcInfoXAry
  Data Store Read3 : DataStoreRead  DataStoreName=DiagcMgrNtcMap
  Data Store Read4 : DataStoreRead  DataStoreName=DiagcMgrNtcInfoXDebCntrAry
  Data Store Write1 : DataStoreWrite  DataStoreName=DiagcMgrNtcInfoXDebCntrAry
  Data Store Write2 : DataStoreWrite  DataStoreName=DiagcMgrNtcInfoXAry
  Selector : Selector  IndexMode=Zero-based  InputPortWidth=22  IndexOptions=Index vector (port)  Indices=[1 3]  OutputSizes=1
  Selector1 : Selector  IndexMode=Zero-based  InputPortWidth=22  IndexOptions=Index vector (port)  Indices=[1 3]  OutputSizes=1
  Selector2 : Selector  IndexMode=Zero-based  InputPortWidth=14  IndexOptions=Index vector (port)  Indices=[1 3]  OutputSizes=1
  Terminator : Terminator
  wires:
  Data Store Read1/1 -> Assignment/1
  Data Store Read3/1 -> Selector1/1
  Constant2/1 -> Assignment1/2
  Selector/1 -> Bus Assignment4/1
  Selector2/1 -> Terminator/1
  NtcInfoIdx/1 -> Assignment/3, Selector/2
  Data Store Read/1 -> Selector/1
  Assignment/1 -> Data Store Write2/1
  Constant1/1 -> Bus Assignment4/3
  Constant4/1 -> Bus Assignment4/4
  Bus Assignment4/1 -> Assignment/2
  Selector1/1 -> Bus Selector3/1
  Constant3/1 -> Bus Assignment4/2
  Data Store Read4/1 -> Assignment1/1, Selector2/1
  Assignment1/1 -> Data Store Write1/1
  Bus Selector3/1 -> Assignment1/3, Selector2/2  "<DebCntrIdx>"
  NtcNr/1 -> Selector1/2

== system ES101A_DiagcMgrProxyX/DiagcMgrProxyApplX/DiagcMgrProxyApplXPer1/Clear All NTCs/Initialize Proxy SetNtc and DiagcData values/Dual Inverter/CopyRight2 ==

== system ES101A_DiagcMgrProxyX/DiagcMgrProxyApplX/DiagcMgrProxyApplXPer1/Clear All NTCs/Initialize Proxy SetNtc and DiagcData values/Dual Inverter1/CopyRight2 ==

== system ES101A_DiagcMgrProxyX/DiagcMgrProxyApplX/DiagcMgrProxyApplXPer1/Clear All NTCs/Initialize Proxy SetNtc and DiagcData values/Single Inverter/CopyRight2 ==

== system ES101A_DiagcMgrProxyX/DiagcMgrProxyApplX/DiagcMgrProxyApplXPer1/Clear All NTCs/Initialize Proxy SetNtc and DiagcData values/Single Inverter1/CopyRight2 ==

== system ES101A_DiagcMgrProxyX/DiagcMgrProxyApplX/DiagcMgrProxyApplXPer1/Update the DiagcSts/For Number of NTCs/Update DiagcSts and Ramp Response/CopyRight2 ==

== system ES101A_DiagcMgrProxyX/DiagcMgrProxyApplX/DiagcMgrProxyApplXPer1/Update the DiagcSts/For Number of NTCs/Update DiagcSts and Ramp Response/Do Nothing ==
  Action Port : ActionPort
  CopyRight2 : Subsystem  Description=|  mask(Copyright Information){none=on}
      | Copyright info block.                                               
      |                                                                     
      | Place copyright information at the top of every subsystem in design.
      mask prompts: none "No parameters"
      mask help: Place copyright information at the top of every subsystem in design.
      mask Display:
      | NxtrConf = 'Nexteer Confidential';
      | 
      | sys = bdroot; %handle for the current model ("system")
      | first = get_param(sys,'Created');
      | first = first(end-3:end);  %year is last four digits
      | 
      | last = get_param(sys,'LastModifiedDate');
      | if isempty(last)
      |     last = datestr(now,'yyyy');
      | else
      |     last = last(end-3:end);
      | end
      | 
      | if strcmp(first,last)
      |     fprintf('%s -- Copyright %s Nexteer',NxtrConf,first)
      | else
      |     fprintf('%s -- %s%s- %s Nexteer',NxtrConf,char(169),first,last)
      | end

== system ES101A_DiagcMgrProxyX/DiagcMgrProxyApplX/DiagcMgrProxyApplXPer1/Update the DiagcSts/For Number of NTCs/Update DiagcSts and Ramp Response/Update Latest Values ==
  NtcNr : Inport
  Action Port : ActionPort
  CopyRight2 : Subsystem  Description=|  mask(Copyright Information){none=on}
      | Copyright info block.                                               
      |                                                                     
      | Place copyright information at the top of every subsystem in design.
      mask prompts: none "No parameters"
      mask help: Place copyright information at the top of every subsystem in design.
      mask Display:
      | NxtrConf = 'Nexteer Confidential';
      | 
      | sys = bdroot; %handle for the current model ("system")
      | first = get_param(sys,'Created');
      | first = first(end-3:end);  %year is last four digits
      | 
      | last = get_param(sys,'LastModifiedDate');
      | if isempty(last)
      |     last = datestr(now,'yyyy');
      | else
      |     last = last(end-3:end);
      | end
      | 
      | if strcmp(first,last)
      |     fprintf('%s -- Copyright %s Nexteer',NxtrConf,first)
      | else
      |     fprintf('%s -- %s%s- %s Nexteer',NxtrConf,char(169),first,last)
      | end
  ProcessDiagcSts : Subsystem  RequirementInfo={} %GIDa_cb335f97_ff4b_4a77_bf67_d4807663aec3  Priority=2
      settings: AttributesFormatString=Priority = %<Priority>
  ProcessRampResponse : Subsystem  RequirementInfo={} %GIDa_7d5e11a5_55eb_408f_85e7_c5c877cacaab  Priority=1
      settings: AttributesFormatString=Priority = %<Priority>
  wires:
  NtcNr/1 -> ProcessRampResponse/1(NtcNr), ProcessDiagcSts/1(NtcNr)

== system ES101A_DiagcMgrProxyX/DiagcMgrProxyApplX/DiagcMgrProxyApplXPer1/Update the DiagcSts/Initialize Proxy Per values/Dual Inverter/CopyRight2 ==

== system ES101A_DiagcMgrProxyX/DiagcMgrProxyApplX/DiagcMgrProxyApplXPer1/Update the DiagcSts/Initialize Proxy Per values/Single Inverter/CopyRight2 ==

== system ES101A_DiagcMgrProxyX/DiagcMgrProxyApplX/DiagcMgrProxyApplXPer1/Update the DiagcSts/Initialize Proxy SetNtc values/Dual Inverter/CopyRight2 ==

== system ES101A_DiagcMgrProxyX/DiagcMgrProxyApplX/DiagcMgrProxyApplXPer1/Update the DiagcSts/Initialize Proxy SetNtc values/Single Inverter/CopyRight2 ==

== system ES101A_DiagcMgrProxyX/DiagcMgrProxyApplX/DiagcMgrProxyApplXPer1/Clear All NTCs/For Number of NTCs in NtcInfoAryX/Clear the NTCs that are active/Do Nothing/CopyRight2 ==

== system ES101A_DiagcMgrProxyX/DiagcMgrProxyApplX/DiagcMgrProxyApplXPer1/Update the DiagcSts/For Number of NTCs/Update DiagcSts and Ramp Response/Do Nothing/CopyRight2 ==

== system ES101A_DiagcMgrProxyX/DiagcMgrProxyApplX/DiagcMgrProxyApplXPer1/Update the DiagcSts/For Number of NTCs/Update DiagcSts and Ramp Response/Update Latest Values/CopyRight2 ==
